simulink model "DC_motor"  (R2015b)
settings: Solver=VariableStepAuto  StartTime=0.0  StopTime=10.0  RelTol=1e-3
undefined symbols (not defined in the file): b, J, K, L, R
settings Model: Creator=mgreiff  LastModifiedBy=mgreiff

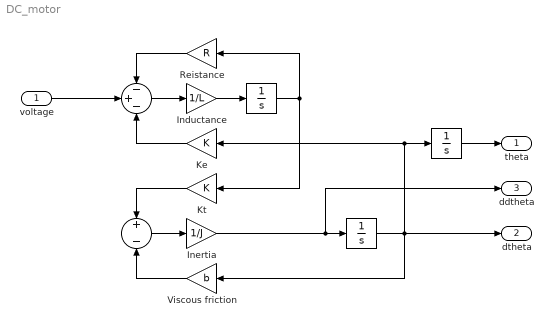
== system DC_motor ==
  voltage : Inport
  " " : Sum  Inputs=-+-
  "  " : Sum  Inputs=+|-
  "   " : Integrator
  "    " : Integrator
  "     " : Integrator
  Inductance : Gain  Gain=1/L
  Inertia : Gain  Gain=1/J
  Ke : Gain  Gain=K
  Kt : Gain  Gain=K
  Reistance : Gain  Gain=R
  Viscous friction : Gain  Gain=b
  theta : Outport
  dtheta : Outport  Port=2
  ddtheta : Outport  Port=3
  wires:
  voltage/1 -> " "/2
  Reistance/1 -> " "/1
  " "/1 -> Inductance/1
  Inductance/1 -> "   "/1
  Ke/1 -> " "/3
  Kt/1 -> "  "/1
  "  "/1 -> Inertia/1
  "   "/1 -> Reistance/1, Kt/1
  Inertia/1 -> ddtheta/1, "    "/1
  "     "/1 -> theta/1
  "    "/1 -> Viscous friction/1, Ke/1, "     "/1, dtheta/1
  Viscous friction/1 -> "  "/2
